simulink model "control_design"  (R2018b)
settings: Solver=FixedStepAuto  StartTime=0.0  StopTime=20  FixedStep=.02  RelTol=1e-3
libraries: simulink x9
settings Model: Creator=Tyler  LastModifiedBy=Tyler

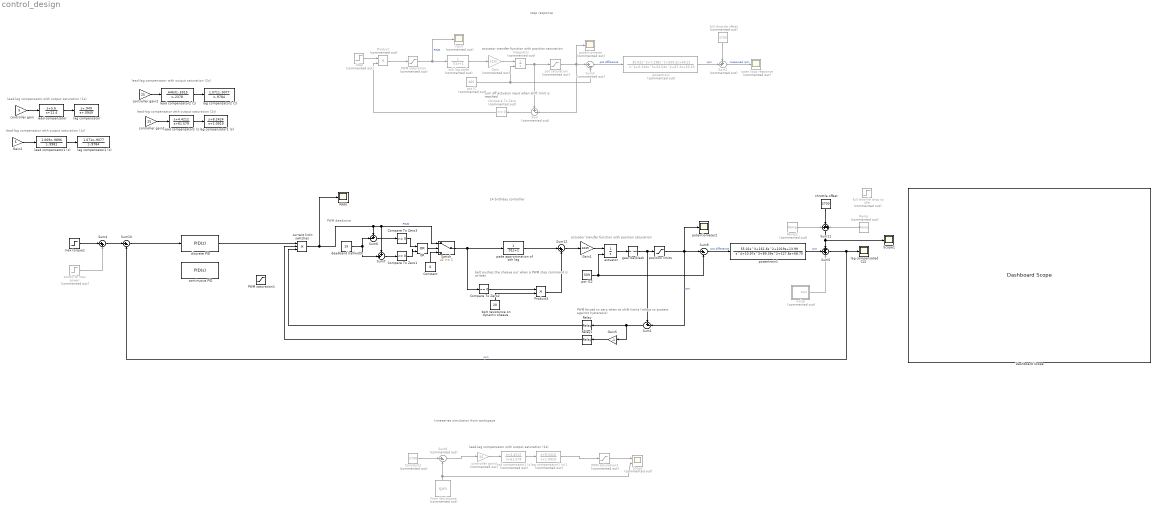
== system control_design ==
  note: PWM deadzone
  note: lead-lag compensator with output saturation (1z)
  note: lead-lag compensator with output saturation (2z)
  note: turn off actuator input
      | when shift limit is reached
  note: actuator transfer function with position saturation
  note: lead-lag compensator with output saturation (1s)
  note: PWM forced to zero when at shift limits
      |  (relays to protect against hysteresis)
  note: actuator transfer function with position saturation
  note: belt pushes the sheave out when a PWM
      | stop command is written
  note: step response
  note: 14 birthday controller
  note: lead-lag compensator with output saturation (2s)
  note: timeseries simulation from workspace
  note: lead-lag compensator with output saturation (2s)
  Compare To Zero : simulink/Logic and Bit Operations/Compare To Zero  Commented=on  relop===  OutDataTypeStr=boolean
  Compare To Zero1 : simulink/Logic and Bit Operations/Compare To Zero  relop=<=  OutDataTypeStr=boolean
  Compare To Zero2 : simulink/Logic and Bit Operations/Compare To Zero  relop===  OutDataTypeStr=boolean
  Compare To Zero3 : simulink/Logic and Bit Operations/Compare To Zero  relop=>=  OutDataTypeStr=boolean
  Constant : Constant  Value=0
  Constant1 : Constant  Commented=on  Value=2700
  Dashboard Scope : DashboardScope  WebBlockId=384
  From Workspace : FromWorkspace  Commented=on  VariableName=rpm  SampleTime=.02  Interpolate=off  OutputAfterFinalValue=Holding final value
  Gain : Gain  Commented=on  Gain=.6239
  Gain1 : Gain  Gain=.6239
  Gain2 : Gain  Gain=5
  Gain5 : Gain  Gain=-1
  Integrator : Integrator  Commented=on  InitialConditionSource=external  InitialCondition=762
  OR : Logic  Operator=OR  IconShape=distinctive  AllPortsSameDT=off  OutDataTypeStr=boolean
  PWM : Scope
  PWM saturation : Saturate  Commented=on  UpperLimit=500  LowerLimit=-500
  PWM saturation1 : Saturate  UpperLimit=500  LowerLimit=-500
  PWM saturation2 : Saturate  Commented=on  UpperLimit=500  LowerLimit=-500
  Product : Product  Commented=on
  Product3 : Product
  Ramp : simulink/Sources/Ramp  Commented=on  slope=3700  start=0  InitialOutput=0
  Ramp1 : simulink/Sources/Ramp  Commented=on  slope=-3700  start=1  InitialOutput=0
  Relay : Relay  OnSwitchValue=1  OffSwitchValue=0  OnOutputValue=0  OffOutputValue=1
  Relay1 : Relay  OnSwitchValue=1  OffSwitchValue=0  OnOutputValue=0  OffOutputValue=1
  Scope : Scope  Commented=on  NumInputPorts=2
  Scope1 : Scope
  Step : Step  Commented=on  Time=0  After=-500  SampleTime=0
  Sum : Sum  Commented=on  Inputs=+-|
  Sum1 : Sum  Inputs=+-|
  Sum10 : Sum  Inputs=|+-
  Sum11 : Sum  Inputs=+++
  Sum12 : Sum  Inputs=|++
  Sum2 : Sum  Commented=on  Inputs=++|
  Sum3 : Sum  Commented=on  Inputs=|+-
  Sum4 : Sum  Inputs=|++
  Sum5 : Sum  Inputs=+++
  Sum6 : Sum  Inputs=+-|
  Sum7 : Sum  Inputs=++|
  Sum8 : Sum  Commented=on  Inputs=|+-
  Sum9 : Sum  Inputs=|+-
  Switch : Switch  Threshold=1
  actuator : Integrator  InitialConditionSource=external  InitialCondition=762  UpperSaturationLimit=460  LowerSaturationLimit=146
  belt resistance on dynamic sheave : Constant  Value=20
  continuous PID : simulink/Continuous/PID Controller  Controller=PID  Form=Parallel  TimeDomain=Continuous-time  SampleTime=-1  IntegratorMethod=Forward Euler  FilterMethod=Forward Euler  ControllerParametersSource=internal  P=24  I=3.84  D=.96  UseFilter=on  N=100  TunerSelectOption=Transfer Function Based (PID Tuner App)  InitialConditionSource=internal  InitialConditionForIntegrator=0  InitialConditionForFilter=0  DifferentiatorICPrevScaledInput=0  ExternalReset=none  TrackingMode=off  Kt=1  LimitOutput=on  UpperSaturationLimit=500  LowerSaturationLimit=-500  LinearizeAsGain=on  AntiWindupMode=clamping  Kb=1  POutMin=[]  POutMax=[]  IOutMin=[]  IOutMax=[]  DOutMin=[]  DOutMax=[]  NOutMin=[]  NOutMax=[]  SumOutMin=[]  SumOutMax=[]  SaturationOutMin=[]  SaturationOutMax=[]  PParamMin=[]  PParamMax=[]  IParamMin=[]  IParamMax=[]  DParamMin=[]  DParamMax=[]  NParamMin=[]  NParamMax=[]  KbParamMin=[]  KbParamMax=[]  KtParamMin=[]  KtParamMax=[]  KbOutMin=[]  KbOutMax=[]  KtOutMin=[]  KtOutMax=[]  IntegratorOutMin=[]  IntegratorOutMax=[]  FilterOutMin=[]  FilterOutMax=[]  SumI1OutMin=[]  SumI1OutMax=[]  SumI2OutMin=[]  SumI2OutMax=[]  SumI3OutMin=[]  SumI3OutMax=[]  SumI4OutMin=[]  SumI4OutMax=[]  SumDOutMin=[]  SumDOutMax=[]  DifferentiatorOutMin=[]  DifferentiatorOutMax=[]  FilterDiffOutCoefMin=[]  FilterDiffOutCoefMax=[]  ReciprocalOutMin=[]  ReciprocalOutMax=[]  SumDenOutMin=[]  SumDenOutMax=[]  SumNumOutMin=[]  SumNumOutMax=[]  DivideOutMin=[]  DivideOutMax=[]  IntegratorContinuousStateAttributes=''  IntegratorStateMustResolveToSignalObject=off  IntegratorRTWStateStorageClass=Auto  FilterContinuousStateAttributes=''  FilterStateMustResolveToSignalObject=off  FilterRTWStateStorageClass=Auto  ParallelPVariant=InternalParameters  IdealPVariant=Disabled  IVariant=InternalParameters  DVariant=InternalParameters  IntegratorVariant=Continuous  SatVariant=Enabled  AWVariant=ContClampingParallel  PCopyVariant=Disabled  TRVariant=Disabled  FdbkBlocksVariant=Forward  IdealPFdbkVariant=Disabled  SatFdbkVariant=Disabled  DerivativeFilterVariant=ContFilter  NVariant=InternalParameters  NCopyVariant=Disabled  FilterICVariant=InternalICsFilter  IntegratorICVariant=InternalICs  ExternalResetVariant=Disabled  TRSumVariant=Passthrough  SumFdbkVariant=Disabled  SumVariant=Sum_PID
  controller gain : Gain  Gain=5
  controller gain1 : Gain  Gain=25
  controller gain2 : Gain  Gain=25
  controller gain3 : Gain  Commented=on  Gain=25
  current limit switches : Product  Inputs=3
  deadband halfwidth : Constant  Value=15
  discrete PID : simulink/Continuous/PID Controller  Controller=PID  Form=Parallel  TimeDomain=Discrete-time  SampleTime=.02  IntegratorMethod=Trapezoidal  FilterMethod=Forward Euler  ControllerParametersSource=internal  P=14  I=2.744  D=.626  UseFilter=on  N=100  TunerSelectOption=Transfer Function Based (PID Tuner App)  InitialConditionSource=internal  InitialConditionForIntegrator=0  InitialConditionForFilter=0  DifferentiatorICPrevScaledInput=0  ExternalReset=none  TrackingMode=off  Kt=1  LimitOutput=on  UpperSaturationLimit=500  LowerSaturationLimit=-500  LinearizeAsGain=on  AntiWindupMode=clamping  Kb=1  POutMin=[]  POutMax=[]  IOutMin=[]  IOutMax=[]  DOutMin=[]  DOutMax=[]  NOutMin=[]  NOutMax=[]  SumOutMin=[]  SumOutMax=[]  SaturationOutMin=[]  SaturationOutMax=[]  PParamMin=[]  PParamMax=[]  IParamMin=[]  IParamMax=[]  DParamMin=[]  DParamMax=[]  NParamMin=[]  NParamMax=[]  KbParamMin=[]  KbParamMax=[]  KtParamMin=[]  KtParamMax=[]  KbOutMin=[]  KbOutMax=[]  KtOutMin=[]  KtOutMax=[]  IntegratorOutMin=[]  IntegratorOutMax=[]  FilterOutMin=[]  FilterOutMax=[]  SumI1OutMin=[]  SumI1OutMax=[]  SumI2OutMin=[]  SumI2OutMax=[]  SumI3OutMin=[]  SumI3OutMax=[]  SumI4OutMin=[]  SumI4OutMax=[]  SumDOutMin=[]  SumDOutMax=[]  DifferentiatorOutMin=[]  DifferentiatorOutMax=[]  FilterDiffOutCoefMin=[]  FilterDiffOutCoefMax=[]  ReciprocalOutMin=[]  ReciprocalOutMax=[]  SumDenOutMin=[]  SumDenOutMax=[]  SumNumOutMin=[]  SumNumOutMax=[]  DivideOutMin=[]  DivideOutMax=[]  IntegratorContinuousStateAttributes=''  IntegratorStateMustResolveToSignalObject=off  IntegratorRTWStateStorageClass=Auto  FilterContinuousStateAttributes=''  FilterStateMustResolveToSignalObject=off  FilterRTWStateStorageClass=Auto  ParallelPVariant=InternalParameters  IdealPVariant=Disabled  IVariant=InternalParameters  DVariant=InternalParameters  IntegratorVariant=Discrete  SatVariant=Enabled  AWVariant=DiscClampingParallel  PCopyVariant=Disabled  TRVariant=Disabled  FdbkBlocksVariant=Feedback  IdealPFdbkVariant=Passthrough  SatFdbkVariant=Passthrough  DerivativeFilterVariant=ForwardEulerFilter  NVariant=InternalParameters  NCopyVariant=Disabled  FilterICVariant=InternalICsFilter  IntegratorICVariant=InternalICs  ExternalResetVariant=Disabled  TRSumVariant=Passthrough  SumFdbkVariant=Enabled  SumVariant=Sum_PID
  full throttle drop to idle : Step  Commented=on  Time=5  After=-2200.  SampleTime=0
  full throttle offset : Constant  Commented=on  Value=3700
  gear backlash : Backlash  BacklashWidth=8
  input : Scope  Commented=on
  lag compensated CLS : Scope
  lag compensator : TransferFcn  Numerator=[1 .949]  Denominator=[1 .0949]
  lag compensator1 (s) : TransferFcn  Numerator=[1 8.2424]  Denominator=[1 1.0919]
  lag compensator1 (s)1 : TransferFcn  Commented=on  Numerator=[1 8.2424]  Denominator=[1 1.0919]
  lag compensator1 (z) : DiscreteTransferFcn  Numerator=[1.071 -.9077]  Denominator=[1 -.9784]
  lag compensator2 (z) : DiscreteTransferFcn  Numerator=[1.071 -.9077]  Denominator=[1 -.9784]
  lead compensator : TransferFcn  Numerator=[1 5.6]  Denominator=[1 11.4]
  lead compensator1 (s) : TransferFcn  Numerator=[1 4.4212]  Denominator=[1 61.579]
  lead compensator1 (s)1 : TransferFcn  Commented=on  Numerator=[1 4.4212]  Denominator=[1 61.579]
  lead compensator1 (z) : DiscreteTransferFcn  Numerator=[1.009 -.9896]  Denominator=[1 -.9981]
  lead compensator2 (z) : DiscreteTransferFcn  Numerator=[.6463 -.5915]  Denominator=[1 -.2378]
  max torque1 : Step  Time=0  After=2700  SampleTime=0
  noise : Subsystem  Commented=on
  open loop response : Scope  Commented=on
  pade approximation of zoh lag : TransferFcn  Denominator=[.01 1]
  position limits : Saturate  UpperLimit=720  LowerLimit=125
  pot IC : Constant  Commented=on  Value=460
  pot IC2 : Constant  Value=509
  pot saturation : Saturate  Commented=on  UpperLimit=460  LowerLimit=146
  potentiometer : Scope  Commented=on
  potentiometer2 : Scope
  powertrain : TransferFcn  Commented=on  Numerator=[35.02 7.238 509.2 49.21]  Denominator=[1 6.234 54.54 87.2 53.23]
  powertrain1 : TransferFcn  Numerator=[55.01 161.6 1019 13.99]  Denominator=[1 10.97 89.39 127.8 68.75]
  switch to max power : Step  Commented=on  Time=4  After=700  SampleTime=0
  throttle offset : Constant  Value=3700
  zoh lag pade : TransferFcn  Commented=on  Denominator=[.01 1]
  wires:
  Sum2/1 -> open loop response/1  "measured rpm"
  full throttle offset/1 -> Sum2/1
  powertrain/1 -> Sum2/2  "rpm"
  Step/1 -> Product/1
  PWM saturation/1 -> input/1, zoh lag pade/1  "PWM"
  Sum5/1 -> Sum10/2, lag compensated CLS/1  "rpm"
  powertrain1/1 -> Sum5/2  "rpm"
  Sum9/1 -> powertrain1/1  "pot difference"
  Sum11/1 -> Scope1/1, Sum5/1
  Product3/1 -> Sum12/2
  belt resistance on dynamic sheave/1 -> Product3/2
  Compare To Zero2/1 -> Product3/1
  Relay1/1 -> current limit switches/2
  Relay/1 -> current limit switches/3
  position limits/1 -> potentiometer2/1, Sum1/2, Sum9/1  "pot"
  Gain5/1 -> Relay1/1
  Sum1/1 -> Gain5/1, Relay/1
  Sum3/1 -> powertrain/1  "pot difference"
  pot IC/1 -> Sum3/2, Integrator/2
  zoh lag pade/1 -> Gain/1
  Gain/1 -> Integrator/1
  Compare To Zero/1 -> Product/2
  pot saturation/1 -> Sum3/1, Sum/2, potentiometer/1
  Integrator/1 -> pot saturation/1, Sum/1
  Sum/1 -> Compare To Zero/1
  lead compensator1 (s)/1 -> lag compensator1 (s)/1
  controller gain1/1 -> lead compensator1 (s)/1
  Sum4/1 -> Sum10/1
  switch to max power/1 -> Sum4/2
  lead compensator2 (z)/1 -> lag compensator2 (z)/1
  controller gain2/1 -> lead compensator2 (z)/1
  controller gain/1 -> lead compensator/1
  lead compensator/1 -> lag compensator/1
  lead compensator1 (z)/1 -> lag compensator1 (z)/1
  Gain2/1 -> lead compensator1 (z)/1
  max torque1/1 -> Sum4/1
  noise/1(Out1) -> Sum5/3
  Gain1/1 -> actuator/1
  pot IC2/1 -> Sum9/2, actuator/2
  actuator/1 -> gear backlash/1
  pade approximation of zoh lag/1 -> Sum12/1
  Sum12/1 -> Gain1/1
  Product/1 -> PWM saturation/1
  Sum6/1 -> Compare To Zero3/1
  Compare To Zero1/1 -> OR/2
  OR/1 -> Switch/2
  Constant/1 -> Switch/3
  Sum7/1 -> Compare To Zero1/1
  deadband halfwidth/1 -> Sum7/2, Sum6/2
  Compare To Zero3/1 -> OR/1
  Switch/1 -> Compare To Zero2/1, pade approximation of zoh lag/1
  current limit switches/1 -> PWM/1, Sum6/1, Sum7/1, Switch/1  "PWM"
  gear backlash/1 -> Sum1/1, position limits/1
  PWM saturation2/1 -> Scope/1
  From Workspace/1 -> Sum8/2, Scope/2
  Constant1/1 -> Sum8/1
  Ramp1/1 -> Sum11/1
  throttle offset/1 -> Sum11/2
  Ramp/1 -> Sum11/3
  controller gain3/1 -> lead compensator1 (s)1/1
  lead compensator1 (s)1/1 -> lag compensator1 (s)1/1
  Sum8/1 -> controller gain3/1
  lag compensator1 (s)1/1 -> PWM saturation2/1
  discrete PID/1 -> current limit switches/1
  Sum10/1 -> discrete PID/1

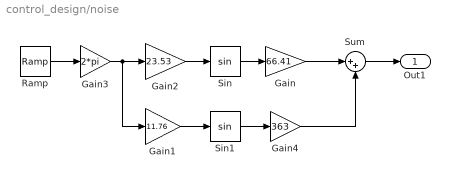
== system control_design/noise ==
  Gain : Gain  Gain=66.41
  Gain1 : Gain  Gain=11.76
  Gain2 : Gain  Gain=23.53
  Gain3 : Gain  Gain=2*pi
  Gain4 : Gain  Gain=363
  Ramp : simulink/Sources/Ramp  slope=1  start=0  InitialOutput=0
  Sin : Trigonometry
  Sin1 : Trigonometry
  Sum : Sum  Inputs=|++
  Out1 : Outport
  wires:
  Ramp/1 -> Gain3/1
  Gain3/1 -> Gain1/1, Gain2/1
  Gain1/1 -> Sin1/1
  Gain2/1 -> Sin/1
  Sin/1 -> Gain/1
  Sin1/1 -> Gain4/1
  Sum/1 -> Out1/1
  Gain/1 -> Sum/1
  Gain4/1 -> Sum/2
